simulink model "SINDYcData"  (R2019a)
settings: Solver=FixedStepAuto  StartTime=0.0  StopTime=Tsim  FixedStep=param.Ts  MaxStep=0.2  RelTol=1e-3
undefined symbols (not defined in the file or in its folder): dist_in, dist_out_1, dist_out_2, F, Fi, param, sigbuilder_block
libraries: simulink x2
settings Model: Creator=yashasvi_sai  LastModifiedBy=ICS
settings SolverCC: ZeroCrossAlgorithm=Adaptive
settings DebuggingCC: IgnoredZcDiagnostic=none

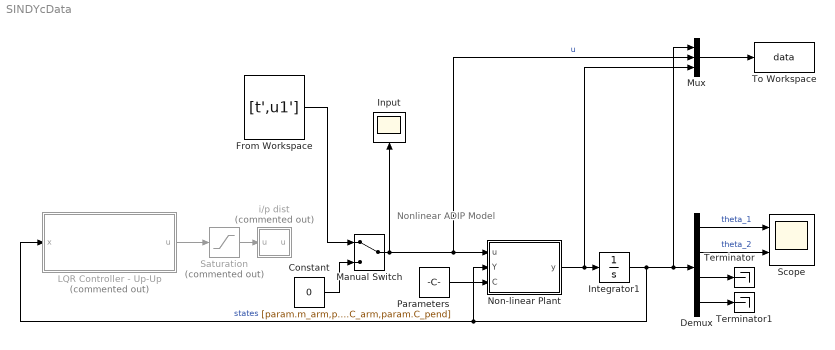
== system SINDYcData ==
  note: Nonlinear ADIP Model
  Constant : Constant  Value=0
  Demux : Demux
  From Workspace : FromWorkspace  VariableName=[t',u1']  SampleTime=0
  Input : Scope
  Integrator1 : Integrator  InitialCondition=param.theta0
  LQR Controller - Up-Up : Subsystem  Commented=on
  Manual Switch : ManualSwitch
  Mux : Mux  Inputs=3
  "Non-linear Plant " : MATLAB Function  TreatAsAtomicUnit=on
  Parameters : Constant  Value=[param.m_arm,param.m_pend,param.m_hinge,param.l_pivot,param.l_pend,param.g,param.Jarm,param.Jpend,param.Jl,param.Jhinge, param.C_arm,param.C_pend]
  Saturation : Saturate  Commented=on  UpperLimit=1.6  LowerLimit=-1.6
  Scope : Scope  NumInputPorts=2
  Terminator : Terminator
  Terminator1 : Terminator
  To Workspace : ToWorkspace  VariableName=data  SampleTime=-1
  i/p dist : Subsystem  Commented=on
  wires:
  LQR Controller - Up-Up/1(u) -> Saturation/1
  Integrator1/1 -> Mux/1, Demux/1, "Non-linear Plant "/2(Y), LQR Controller - Up-Up/1(x)  "states"
  Parameters/1 -> "Non-linear Plant "/3(C)
  Demux/4 -> Terminator1/1
  Demux/3 -> Terminator/1
  Demux/1 -> Scope/1  "theta_1"
  Demux/2 -> Scope/2  "theta_2"
  Manual Switch/1 -> Mux/2, "Non-linear Plant "/1(u), Input/1  "u"
  Constant/1 -> Manual Switch/2
  Mux/1 -> To Workspace/1
  Saturation/1 -> i/p dist/1(u)
  From Workspace/1 -> Manual Switch/1
  "Non-linear Plant "/1(y) -> Mux/3, Integrator1/1

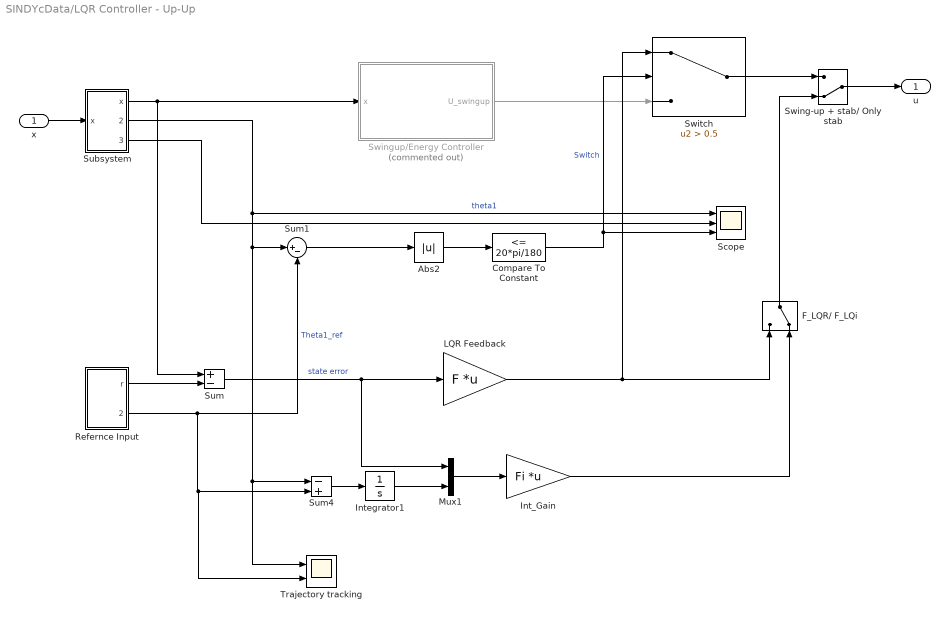
== system SINDYcData/LQR Controller - Up-Up ==
  x : Inport
  Abs2 : Abs
  Compare To Constant : simulink/Logic and Bit Operations/Compare To Constant  relop=<=  const=20*pi/180  OutDataTypeStr=boolean
  F_LQR/ F_LQi : ManualSwitch  CurrentSetting=0
  Int_Gain : Gain  Gain=Fi  Multiplication=Matrix(K*u)
  Integrator1 : Integrator
  LQR Feedback : Gain  Gain=F  Multiplication=Matrix(K*u)
  Mux1 : Mux  Inputs=2
  Refernce Input : Subsystem
  Scope : Scope  NumInputPorts=3
  Subsystem : Subsystem
  Sum : Sum  Inputs=+-
  Sum1 : Sum  Inputs=|+-
  Sum4 : Sum  Inputs=-+
  "Swing-up + stab/ Only stab " : ManualSwitch  CurrentSetting=0
  Swingup/Energy Controller : Subsystem  Commented=on
  Switch : Switch  Criteria=u2 > Threshold  Threshold=0.5
  Trajectory tracking : Scope  NumInputPorts=2
  u : Outport
  wires:
  Switch/1 -> "Swing-up + stab/ Only stab "/1
  Swingup/Energy Controller/1(U_swingup) -> Switch/3
  Refernce Input/1(r) -> Sum/2
  Abs2/1 -> Compare To Constant/1
  Compare To Constant/1 -> Scope/3, Switch/2  "Switch"
  Sum1/1 -> Abs2/1
  LQR Feedback/1 -> F_LQR/ F_LQi/1, Switch/1
  "Swing-up + stab/ Only stab "/1 -> u/1
  Sum/1 -> LQR Feedback/1, Mux1/1  "state error"
  Integrator1/1 -> Mux1/2
  Refernce Input/2(theta1ref) -> Trajectory tracking/2, Sum4/2, Sum1/2  "Theta1_ref"
  Mux1/1 -> Int_Gain/1
  F_LQR/ F_LQi/1 -> "Swing-up + stab/ Only stab "/2
  Int_Gain/1 -> F_LQR/ F_LQi/2
  Sum4/1 -> Integrator1/1
  Subsystem/1("x ") -> Sum/1, Swingup/Energy Controller/1(x)
  Subsystem/2(theta1) -> Sum4/1, Trajectory tracking/1, Sum1/1, Scope/1  "theta1"
  x/1 -> Subsystem/1(x)
  Subsystem/3(theta2) -> Scope/2

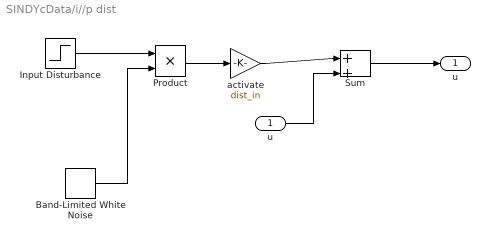
== system SINDYcData/i//p dist ==
  u : Inport
  Band-Limited White Noise : simulink/Sources/Band-Limited White Noise  Cov=[0.08]  Ts=0.1  seed=[23341]
  Input Disturbance : Step  After=0.05  SampleTime=0
  Product : Product
  Sum : Sum  Inputs=|++
  activate : Gain  Gain=dist_in
  " u " : Outport
  wires:
  activate/1 -> Sum/1
  u/1 -> Sum/2
  Sum/1 -> " u "/1
  Input Disturbance/1 -> Product/1
  Product/1 -> activate/1
  Band-Limited White Noise/1 -> Product/2

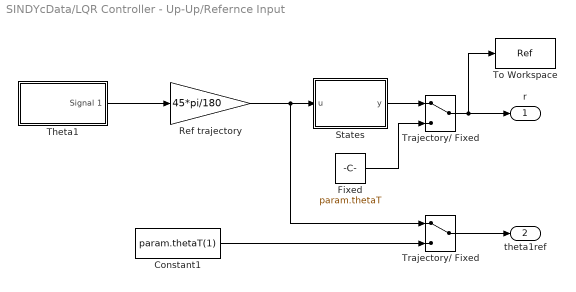
== system SINDYcData/LQR Controller - Up-Up/Refernce Input ==
  Constant1 : Constant  Value=param.thetaT(1)
  Fixed : Constant  Value=param.thetaT
  Ref trajectory : Gain  Gain=45*pi/180
  States : MATLAB Function  TreatAsAtomicUnit=on
  Theta1 : Subsystem  Tag=STV Subsys  LoadFcn=sigbuilder_block('load');  StartFcn=sigbuilder_block('start');  StopFcn=sigbuilder_block('stop');  ClipboardFcn=sigbuilder_block('clipboard');  mask(Sigbuilder block){tuvar=[0:10]}
      mask help: Simulink:masks:SigbuilderBlock_MD
      mask init:
      | if ~strcmp(get_param(bdroot(gcbh),'SimulationStatus'),'stopped') tuvar = sigbuilder_block('maskInit'); end
      settings: CopyFcn=sigbuilder_block('copy');  DeleteFcn=sigbuilder_block('delete');  ModelCloseFcn=sigbuilder_block('modelClose');  PreSaveFcn=sigbuilder_block('preSave');  PauseFcn=sigbuilder_block('pause');  ContinueFcn=sigbuilder_block('continue');  NameChangeFcn=sigbuilder_block('namechange');  OpenFcn=sigbuilder_block('open',[5.4 30 1141.2 522.6 ]);  CloseFcn=sigbuilder_block('close');
      mask Display: plot(0, 0, 100, 100,[2, 2, 32, 32, 2], [68, 8, 8, 68, 68],[32, 2], [38, 38], [32, 19, 2],[53, 60, 44], [32, 17, 17, 2],[16, 16, 31, 31]);txt = getActiveGroup(gcbh);text(2, 100, txt,'verticalAlignment', 'top');
  To Workspace : ToWorkspace  VariableName=Ref  SampleTime=-1
  Trajectory/ Fixed : ManualSwitch
  Trajectory/ Fixed : ManualSwitch
  r : Outport
  theta1ref : Outport  Port=2
  wires:
  States/1(y) -> Trajectory/ Fixed/1
  Fixed/1 -> Trajectory/ Fixed/2
  Trajectory/ Fixed/1 -> To Workspace/1, r/1
  Constant1/1 -> Trajectory/ Fixed/2
  Trajectory/ Fixed/1 -> theta1ref/1
  Ref trajectory/1 -> Trajectory/ Fixed/1, States/1(u)
  Theta1/1(Signal 1) -> Ref trajectory/1

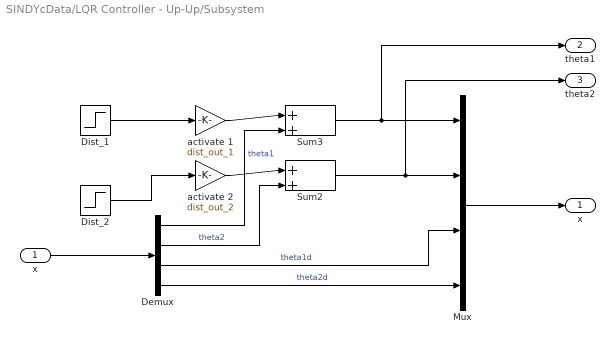
== system SINDYcData/LQR Controller - Up-Up/Subsystem ==
  x : Inport
  Demux : Demux
  Dist_1 : Step  Time=30  After=0.1  SampleTime=0
  Dist_2 : Step  Time=20  After=0.05  SampleTime=0
  Mux : Mux
  Sum2 : Sum  Inputs=|++
  Sum3 : Sum  Inputs=|++
  activate 1 : Gain  Gain=dist_out_1
  activate 2 : Gain  Gain=dist_out_2
  "x " : Outport
  theta1 : Outport  Port=2
  theta2 : Outport  Port=3
  wires:
  Sum3/1 -> theta1/1, Mux/1
  Demux/2 -> Sum2/2  "theta2"
  Sum2/1 -> theta2/1, Mux/2
  Demux/3 -> Mux/3  "theta1d"
  Demux/1 -> Sum3/2  "theta1"
  activate 2/1 -> Sum2/1
  x/1 -> Demux/1
  Dist_2/1 -> activate 2/1
  Demux/4 -> Mux/4  "theta2d"
  activate 1/1 -> Sum3/1
  Mux/1 -> "x "/1
  Dist_1/1 -> activate 1/1

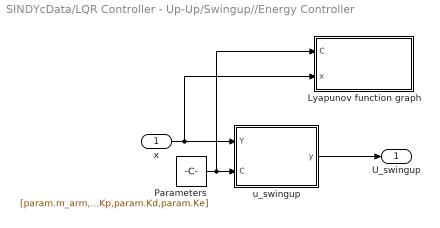
== system SINDYcData/LQR Controller - Up-Up/Swingup//Energy Controller ==
  x : Inport
  Lyapunov function graph : Subsystem
  Parameters : Constant  Value=[param.m_arm,param.m_pend,param.m_hinge,param.l_pivot,param.l_pend,param.g,param.Jarm,param.Jpend,param.Jl,param.Jhinge, param.C_arm,param.C_pend,param.Kp,param.Kd,param.Ke]
  "u_swingup " : MATLAB Function  TreatAsAtomicUnit=on
  U_swingup : Outport
  wires:
  x/1 -> Lyapunov function graph/2(x), "u_swingup "/1(Y)
  Parameters/1 -> Lyapunov function graph/1(C), "u_swingup "/2(C)
  "u_swingup "/1(y) -> U_swingup/1

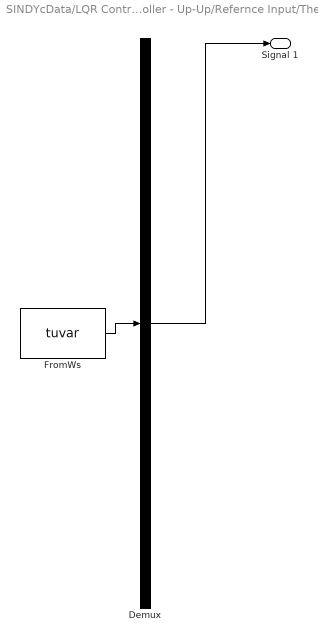
== system SINDYcData/LQR Controller - Up-Up/Refernce Input/Theta1 ==
  Demux : Demux  Tag=STV Demux  Outputs=1
  FromWs : FromWorkspace  Tag=STV FromWs  VariableName=tuvar  SampleTime=0
      SigBuilderData=|
      | common.afterFinalStr = 'Extrapolate'
      | common.sampleTime = 0
      | dataSet.timeRange = [0 50]
      | dataSet.name = 'Group 1'
      | sbobj.Groups.Name = 'Group 1'
      | sbobj.Groups.Signals.Name = 'Signal 1'
      | sbobj.Groups.Signals.XData = [0 3 5 7 9 11 13 40 50]
      | sbobj.Groups.Signals.YData = [0 0 1 1 -1 -1 0 0 0]
      | sbobj.Groups.TimeRange = [0 50]
  Signal 1 : Outport  Tag=STV Outport
  wires:
  Demux/1 -> Signal 1/1
  FromWs/1 -> Demux/1

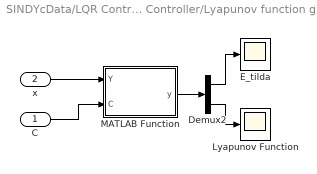
== system SINDYcData/LQR Controller - Up-Up/Swingup//Energy Controller/Lyapunov function graph ==
  C : Inport
  x : Inport  Port=2
  Demux2 : Demux  Outputs=2
  E_tilda : Scope
  Lyapunov Function : Scope
  MATLAB Function : MATLAB Function  TreatAsAtomicUnit=on
  wires:
  Demux2/1 -> E_tilda/1
  MATLAB Function/1(y) -> Demux2/1
  C/1 -> MATLAB Function/2(C)
  Demux2/2 -> Lyapunov Function/1
  x/1 -> MATLAB Function/1(Y)

== matlab function SINDYcData/LQR Controller - Up-Up/Swingup//Energy Controller/u_swingup  ==
  data: Y input; y output; C input
function y = fcn(Y, C)
m1=C(1); % Mass of arm
m2=C(2); % Mass of pendulum
mh = C(3); % Mass of Hinge
l1  = C(4); % Length of arm
l2 = C(5); % Length of pendulum
g_ = C(6);
J_arm = C(7);
J_pend = C(8);
J_motor = C(9);
J_sensor = C(10);
fv1 = C(11);
fv2 = C(12);

y1 = Y(1);  % actual theta1          
y2 = Y(2);  % actual theta2
y3 = Y(3);  % actual theta1d
y4 = Y(4);  % actual theta2d

Kp = C(13);
Kd = C(14);
Ke = C(15);

y1_tilda = Y(1) - pi;

u_swing = -(Kd*((g_*l1*l2^2*m2^2*sin(y1))/8 - (fv1*l2^2*m2*y3)/4 - (l1^2*l2^2*m2^2*y3^2*sin(2*y1 - 2*y2))/8 - (l1*l2^3*m2^2*y4^2*sin(y1 - y2))/8 - J_pend*fv1*y3 + (J_pend*g_*l1*m1*sin(y1))/2 + J_pend*g_*l1*m2*sin(y1) + J_pend*g_*l1*mh*sin(y1) + (g_*l1*l2^2*m2^2*sin(y1 - 2*y2))/8 + (fv2*l1*l2*m2*y4*cos(y1 - y2))/2 + (g_*l1*l2^2*m1*m2*sin(y1))/8 + (g_*l1*l2^2*m2*mh*sin(y1))/4 - (J_pend*l1*l2*m2*y4^2*sin(y1 - y2))/2) + (y3 + Kp*y1_tilda)*(J_arm*J_pend + J_motor*J_pend + J_pend*J_sensor + (l1^2*l2^2*m2^2)/4 + (J_arm*l2^2*m2)/4 + (J_motor*l2^2*m2)/4 + (J_pend*l1^2*m1)/4 + J_pend*l1^2*m2 + (J_sensor*l2^2*m2)/4 - (l1^2*l2^2*m2^2*cos(y1 - y2)^2)/4 + (l1^2*l2^2*m1*m2)/16))/(Kd*((m2*l2^2)/4 + J_pend) + Ke*((J_arm*y3^2)/2 + (J_motor*y3^2)/2 + (J_pend*y4^2)/2 + (J_sensor*y3^2)/2 - g_*m1*(l1/2 - (l1*cos(y1))/2) - g_*m2*(l1 + l2/2 - l1*cos(y1) - (l2*cos(y2))/2) - g_*mh*(l1 - l1*cos(y1)) - 6321319090251713/9007199254740992)*(J_arm*J_pend + J_motor*J_pend + J_pend*J_sensor + (l1^2*l2^2*m2^2)/4 + (J_arm*l2^2*m2)/4 + (J_motor*l2^2*m2)/4 + (J_pend*l1^2*m1)/4 + J_pend*l1^2*m2 + (J_sensor*l2^2*m2)/4 - (l1^2*l2^2*m2^2*cos(y1 - y2)^2)/4 + (l1^2*l2^2*m1*m2)/16));

y = u_swing;

== matlab function SINDYcData/Non-linear Plant  ==
  data: u input; Y input; y output; C input
function y = fcn(u,Y,C)
m1=C(1); % Mass of arm
m2=C(2); % Mass of pendulum
mh = C(3); % Mass of Hinge
l1  = C(4); % Length of arm
l2 = C(5); % Length of pendulum
g_ = C(6);
J_arm = C(7);
J_pend = C(8);
J_motor = C(9);
J_sensor = C(10);
fv1 = C(11);
fv2 = C(12);

y1 = Y(1);  % actual theta1          
y2 = Y(2);  % actual theta2
y3 = Y(3);  % actual theta1d
y4 = Y(4);  % actual theta2d

dy1 = y3;
dy2 = y4;
dy3 =-(2*(8*J_pend*fv1*y3 - 2*l2^2*m2*u - 8*J_pend*u + 2*fv1*l2^2*m2*y3 + l1^2*l2^2*m2^2*y3^2*sin(2*y1 - 2*y2) + l1*l2^3*m2^2*y4^2*sin(y1 - y2) + g_*l1*l2^2*m2^2*sin(y1) + 4*J_pend*g_*l1*m1*sin(y1) + 8*J_pend*g_*l1*m2*sin(y1) + 8*J_pend*g_*l1*mh*sin(y1) + g_*l1*l2^2*m2^2*sin(y1 - 2*y2) - 4*fv2*l1*l2*m2*y4*cos(y1 - y2) + g_*l1*l2^2*m1*m2*sin(y1) + 2*g_*l1*l2^2*m2*mh*sin(y1) + 4*J_pend*l1*l2*m2*y4^2*sin(y1 - y2)))/(16*J_arm*J_pend + 16*J_motor*J_pend + 16*J_pend*J_sensor + 4*l1^2*l2^2*m2^2 + 4*J_arm*l2^2*m2 + 4*J_motor*l2^2*m2 + 4*J_pend*l1^2*m1 + 16*J_pend*l1^2*m2 + 4*J_sensor*l2^2*m2 - 4*l1^2*l2^2*m2^2*cos(y1 - y2)^2 + l1^2*l2^2*m1*m2);
dy4 =(2*(l1^2*l2^2*m2^2*y4^2*sin(2*y1 - 2*y2) - 8*J_motor*fv2*y4 - 8*J_sensor*fv2*y4 - 2*fv2*l1^2*m1*y4 - 8*fv2*l1^2*m2*y4 - 8*J_arm*fv2*y4 - 4*l1*l2*m2*u*cos(y1 - y2) + 2*g_*l1^2*l2*m2^2*sin(2*y1 - y2) + 4*l1^3*l2*m2^2*y3^2*sin(y1 - y2) - 2*g_*l1^2*l2*m2^2*sin(y2) - 4*J_arm*g_*l2*m2*sin(y2) - 4*J_motor*g_*l2*m2*sin(y2) - 4*J_sensor*g_*l2*m2*sin(y2) + g_*l1^2*l2*m1*m2*sin(2*y1 - y2) + 2*g_*l1^2*l2*m2*mh*sin(2*y1 - y2) + l1^3*l2*m1*m2*y3^2*sin(y1 - y2) + 4*fv1*l1*l2*m2*y3*cos(y1 - y2) + 2*g_*l1^2*l2*m2*mh*sin(y2) + 4*J_arm*l1*l2*m2*y3^2*sin(y1 - y2) + 4*J_motor*l1*l2*m2*y3^2*sin(y1 - y2) + 4*J_sensor*l1*l2*m2*y3^2*sin(y1 - y2)))/(16*J_arm*J_pend + 16*J_motor*J_pend + 16*J_pend*J_sensor + 2*l1^2*l2^2*m2^2 + 4*J_arm*l2^2*m2 + 4*J_motor*l2^2*m2 + 4*J_pend*l1^2*m1 + 16*J_pend*l1^2*m2 + 4*J_sensor*l2^2*m2 - 2*l1^2*l2^2*m2^2*cos(2*y1 - 2*y2) + l1^2*l2^2*m1*m2);
y = [dy1 dy2 dy3 dy4]';

== matlab function SINDYcData/LQR Controller - Up-Up/Swingup//Energy Controller/Lyapunov function graph/MATLAB Function ==
  data: Y input; y output; C input
function y = fcn(Y,C)

m1=C(1); % Mass of arm
m2=C(2); % Mass of pendulum
mh = C(3); % Mass of Hinge
l1  = C(4); % Length of arm
l2 = C(5); % Length of pendulum
g_ = C(6);
J_arm = C(7);
J_pend = C(8);
J_motor = C(9);
J_sensor = C(10);
fv1 = C(11);
fv2 = C(12);

y1 = Y(1);  % actual theta1          
y2 = Y(2);  % actual theta2
y3 = Y(3);  % actual theta1d
y4 = Y(4);  % actual theta2d

Kp = C(13);
Kd = C(14);
Ke = C(15);

y1_tilda = Y(1) - pi;

E_tilda = (J_arm*y3^2)/2 + (J_motor*y3^2)/2 + (J_pend*y4^2)/2 + (J_sensor*y3^2)/2 + g_*m1*(l1/2 - (l1*cos(y1))/2) + g_*m2*(l1 + l2/2 - l1*cos(y1) - (l2*cos(y2))/2) + g_*mh*(l1 - l1*cos(y1)) - 6321319090251713/9007199254740992;
V_L = 0.5*(Ke*E_tilda^2 + Kd*y3^2 + Kp*(y1_tilda)^2);

y = [E_tilda V_L];

== matlab function SINDYcData/LQR Controller - Up-Up/Refernce Input/States ==
  data: u input; y output
function y = fcn(u)
r = [u;0;0;0];
y = r;
